simulink model "PLANTA_COMPLETA"  (R2024b)
settings: Solver=FixedStepAuto  StartTime=0.0  StopTime=inf  FixedStep=0.001  MaxStep=0.0005  RelTol=1e-4
undefined symbols (not defined in the file): A_hm, A_tm, at_breakpoints, at_max, b_ha, B_hm, b_ta, B_tm, bcx, bcy, bhd, bhEb, bhm, bt, btd, btm, btw, bwu, C_hm, C_tm, D_hm, D_tm, DiscIntNeverNeededParam, dl_h_ini, dx_l_ini, dx_t_ini, dx_td_ini, dxt_max, dy_l_ini, F01_a_t_max, F01_Ts1, F02_a_h_max, F02_Ts1, F03_a_h_max, F03_a_t_max, F03_dxt_max, F03_Ts1, Fhw_min, g, Hc, ih, it, Jhd_hEb, Jhm_hb, Jtd, Jtm_tb, K_hsa, K_hsia, K_tsa, K_tsia, Kcy, Kd_table, Ke_tita, Ke_w, kp_pos, Kp_table, kp_w, Ktw, kwu, l_breakpoints ... (+30)
libraries: simulink x13, spsEdgeDetectorLib x5, simulink_extras x2, dspsigops x2, vrlib x1, dspstat3 x1
(part 4 of 5)

== system PLANTA_COMPLETA/Nivel 2 - Control Regulatorio + Obs/Observador_Control_Posicion/Fuerzas de tension de cable en Carro ==
  x_td : Inport
  dx_td : Inport  Port=2
  x_t : Inport  Port=3
  dx_t : Inport  Port=4
  Add : Sum  Inputs=+-
  Add1 : Sum  Inputs=+-
  Add2 : Sum
  Gain : Gain  Gain=Ktw
  Gain1 : Gain  Gain=btw
  F_tw : Outport
  wires:
  Add1/1 -> Gain1/1
  Add/1 -> Gain/1
  Gain1/1 -> Add2/2
  x_td/1 -> Add/1
  dx_t/1 -> Add1/2
  dx_td/1 -> Add1/1
  Gain/1 -> Add2/1
  Add2/1 -> F_tw/1
  x_t/1 -> Add/2

== system PLANTA_COMPLETA/Nivel 2 - Control Regulatorio + Obs/Observador_Control_Posicion/Observador ==
  x_td : Inport
  T_tm* : Inport  Port=2
  Discrete-Time Integrator : DiscreteIntegrator  InitialCondition=x_td_ini  SampleTime=T_s2  ICPrevOutput=DiscIntNeverNeededParam  ICPrevScaledInput=DiscIntNeverNeededParam
  Discrete-Time Integrator1 : DiscreteIntegrator  InitialCondition=dx_td_ini  SampleTime=T_s2  ICPrevOutput=DiscIntNeverNeededParam  ICPrevScaledInput=DiscIntNeverNeededParam
  Gain : Gain  Gain=rtd/(Jtd+Jtm_tb*(it)^2)
  Gain1 : Gain  Gain=Ke_tita
  Gain2 : Gain  Gain=Ke_w
  Gain3 : Gain  Gain=it
  Scope : Scope  NumInputPorts=3
  Sum1 : Sum  Inputs=|++
  Sum2 : Sum  Inputs=|++
  Sum3 : Sum  Inputs=+-|
  dx_td_obs : Outport
  wires:
  T_tm*/1 -> Gain3/1
  Gain/1 -> Sum1/1
  Sum1/1 -> Discrete-Time Integrator1/1  "ddx_td_obs"
  x_td/1 -> Scope/1, Sum3/1
  Sum3/1 -> Gain2/1, Gain1/1
  Gain1/1 -> Sum2/2
  Gain2/1 -> Sum1/2
  Sum2/1 -> Scope/3, Discrete-Time Integrator/1, dx_td_obs/1
  Gain3/1 -> Gain/1
  Discrete-Time Integrator/1 -> Scope/2, Sum3/2
  Discrete-Time Integrator1/1 -> Sum2/1

== system PLANTA_COMPLETA/Nivel 2 - Control Regulatorio + Obs/Observador_Control_Posicion/Subsystem ==
  xt_obs : Inport
  xt_ref : Inport  Port=2
  Discrete Derivative : simulink/Discrete/Discrete Derivative  Commented=on  gainval=1.0  ICPrevScaledInput=0.0  OutMin=[]  OutMax=[]  OutDataType=fixdt(1, 16)  OutScaling=2^-10  DoSatur=off
  Gain : Gain  Gain=kp_pos
  Gain1 : Gain  Commented=on  Gain=kp_w
  Sum : Sum  Inputs=|++
  Sum1 : Sum  Inputs=|-+
  dxt_pos : Outport
  wires:
  xt_ref/1 -> Sum1/2
  Sum1/1 -> Discrete Derivative/1, Gain/1
  Gain/1 -> Sum/1  "dxt_pos"
  Gain1/1 -> Sum/2  "dxt_pos"
  Sum/1 -> dxt_pos/1
  xt_obs/1 -> Sum1/1
  Discrete Derivative/1 -> Gain1/1

== system PLANTA_COMPLETA/Nivel 2 - Control Regulatorio + Obs/Observador_Control_Posicion/Traslacion del carro ==
  F_tw : Inport
  F_hw : Inport  Port=2
  theta_l : Inport  Port=3
  Discrete-Time Integrator : DiscreteIntegrator  InitialCondition=dx_t_ini  SampleTime=T_s2  ICPrevOutput=DiscIntNeverNeededParam  ICPrevScaledInput=DiscIntNeverNeededParam
  Discrete-Time Integrator1 : DiscreteIntegrator  InitialCondition=x_t_ini  SampleTime=T_s2  ICPrevOutput=DiscIntNeverNeededParam  ICPrevScaledInput=DiscIntNeverNeededParam
  Gain : Gain  Gain=2
  Gain1 : Gain  Gain=bt
  Gain2 : Gain  Gain=1/Mt
  Product : Product
  Sin : Trigonometry
  Sum : Sum  Inputs=++-
  x_t : Outport
  dx_t : Outport  Port=2
  wires:
  Gain1/1 -> Sum/3
  theta_l/1 -> Sin/1
  Sin/1 -> Product/2
  Sum/1 -> Gain2/1
  F_tw/1 -> Sum/1
  F_hw/1 -> Product/1
  Gain/1 -> Sum/2
  Product/1 -> Gain/1
  Gain2/1 -> Discrete-Time Integrator/1  "ddx_t"
  Discrete-Time Integrator/1 -> Discrete-Time Integrator1/1, Gain1/1, dx_t/1
  Discrete-Time Integrator1/1 -> x_t/1

== system PLANTA_COMPLETA/PLANTA/ACC DE CARRO/Freno ==
  dx_td : Inport
  BRK_t : Inport  Port=2
  Constant : Constant  Value=0
  Gain4 : Gain  Gain=-(btd*it)/rtd
  Saturation : Saturate  UpperLimit=Ttb_Max  LowerLimit=-Ttb_Max
  Switch : Switch  Criteria=u2 ~= 0  SaturateOnIntegerOverflow=off  InputSameDT=off
  T_tb : Outport
  wires:
  Constant/1 -> Switch/1
  BRK_t/1 -> Switch/2
  Saturation/1 -> Switch/3
  Switch/1 -> T_tb/1  "T_tb"
  Gain4/1 -> Saturation/1
  dx_td/1 -> Gain4/1

== system PLANTA_COMPLETA/PLANTA/ACC DE IZAJE/Freno ==
  w_hm : Inport
  BRK_h : Inport  Port=2
  Constant : Constant  Value=0
  Gain5 : Gain  Gain=-bhd
  Saturation : Saturate  UpperLimit=Thb_Max  LowerLimit=-Thb_Max
  Switch : Switch  Criteria=u2 ~= 0  SaturateOnIntegerOverflow=off  InputSameDT=off
  T_hb : Outport
  wires:
  Gain5/1 -> Saturation/1
  BRK_h/1 -> Switch/2
  Saturation/1 -> Switch/3
  Constant/1 -> Switch/1
  w_hm/1 -> Gain5/1
  Switch/1 -> T_hb/1

== system PLANTA_COMPLETA/PLANTA/ACC DE IZAJE/Freno Emergencia ==
  w_hd : Inport
  BRK_hE : Inport  Port=2
  Constant : Constant  Value=0
  Gain5 : Gain  Gain=-bhEb
  Saturation : Saturate  UpperLimit=ThEb_Max  LowerLimit=-ThEb_Max
  Switch : Switch  Criteria=u2 ~= 0  SaturateOnIntegerOverflow=off  InputSameDT=off
  T_hEB : Outport
  wires:
  Gain5/1 -> Saturation/1
  BRK_hE/1 -> Switch/2
  Saturation/1 -> Switch/3
  Constant/1 -> Switch/1
  w_hd/1 -> Gain5/1
  Switch/1 -> T_hEB/1

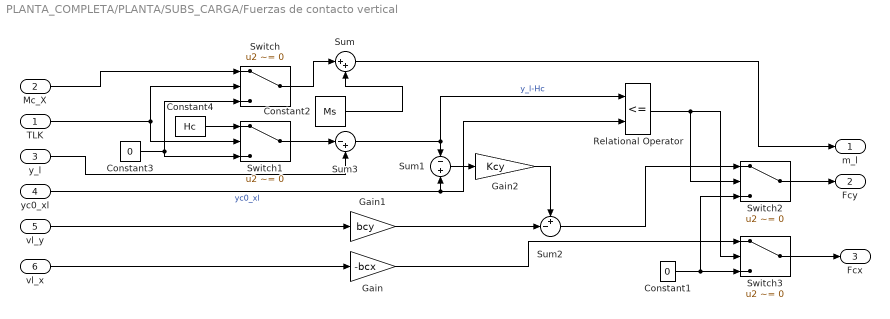
== system PLANTA_COMPLETA/PLANTA/SUBS_CARGA/Fuerzas de contacto vertical ==
  TLK : Inport
  Mc_X : Inport  Port=2
  y_l : Inport  Port=3
  yc0_xl : Inport  Port=4
  vl_y : Inport  Port=5
  vl_x : Inport  Port=6
  Constant1 : Constant  Value=0
  Constant2 : Constant  Value=Ms
  Constant3 : Constant  Value=0
  Constant4 : Constant  Value=Hc
  Gain : Gain  Gain=-bcx
  Gain1 : Gain  Gain=bcy
  Gain2 : Gain  Gain=Kcy
  Relational Operator : RelationalOperator  Operator=<=  OutDataTypeStr=boolean  RndMeth=Simplest  InputSameDT=off
  Sum : Sum  Inputs=|++
  Sum1 : Sum  Inputs=-|+
  Sum2 : Sum  Inputs=+-|
  Sum3 : Sum  Inputs=|-+
  Switch{,1..3} (4 alike) : Switch  Criteria=u2 ~= 0  SaturateOnIntegerOverflow=off  InputSameDT=off
  m_l : Outport
  Fcy : Outport  Port=2
  Fcx : Outport  Port=3
  wires:
  TLK/1 -> Switch/2, Switch1/2
  Gain1/1 -> Sum2/2
  Switch/1 -> Sum/1
  Constant3/1 -> Switch1/3, Switch/3
  Constant2/1 -> Sum/2
  Sum2/1 -> Switch2/1
  vl_y/1 -> Gain1/1
  Gain/1 -> Switch3/1
  Constant4/1 -> Switch1/1
  vl_x/1 -> Gain/1
  Gain2/1 -> Sum2/1
  Sum1/1 -> Gain2/1
  Sum/1 -> m_l/1
  Mc_X/1 -> Switch/1
  Constant1/1 -> Switch3/3, Switch2/3
  Relational Operator/1 -> Switch3/2, Switch2/2
  Sum3/1 -> Sum1/1, Relational Operator/1  "y_l-Hc"
  Switch1/1 -> Sum3/1
  y_l/1 -> Sum3/2
  Switch2/1 -> Fcy/1
  Switch3/1 -> Fcx/1
  yc0_xl/1 -> Relational Operator/2, Sum1/2  "yc0_xl"

== matlab function PLANTA_COMPLETA/PLANTA/PERFIL_OBSTACULOS/sensor ==
  data: y0_array input; distancia output; index input; Yt0 parameter
function distancia= mideDistancia(y0_array,index, Yt0)
distancia = Yt0-y0_array(index);

== matlab function PLANTA_COMPLETA/PLANTA/Altura perfil obstaculos (A partir de posicion x_l)/Calculo ==
  data: y0_array input; yc0_xt output; index input
function yc0_xt= calcula_y0(y0_array,index)

if (index>0 && index<=32)
    yc0_xt =y0_array(index);
else
    yc0_xt=0;    
end

== stateflow chart PLANTA_COMPLETA/Nivel 1 - Control Supervisor ==
  state PERFIL_DE_OBSTACULOS [parallel]
    entry:
    num_index = floor(80/Wc);
    Y_perfil = zeros(1,num_index,'double');
    during:
    %xtd = theta_mt*pulsos_x_rev*dist_x_pulso*(1/100);
    xtd_lidar = (xtd+30)+3;
    index = floor(xtd_lidar/Wc);
    Y_c0_read = yc0_xt;
    if index>0 && index<=32
    Y_perfil(index) = Y_c0_read;
    end
    settings: executionOrder=2
  state OFF [parallel]
    settings: executionOrder=1
    state EMERGENCIA
      entry:
      %Cuando el control supervisor entra en esta de emergencia, cede
      %el control al Nivel 0 hasta retomar el estado normal
      dxt_ref=0;
      dlh_ref=0;
      ddxt_ref=0;
    state ON
      entry:
      dxt_ref_ant = 0;
      dlh_ref_ant = 0;
      dxt_ref = 0;
      dlh_ref = 0;
      ddxt_ref = 0;
      state DETECCION_ESTADOS [parallel]
        settings: executionOrder=1
        state TWISTLOCKS [parallel]
          settings: executionOrder=1
          state VERIFICAR
          state ACT_TLK
            entry:
            TLK=1;
            c=-ceil((xtd+30)/Wc);
            during:
            y_real=45-(lh+Hc);
          state DES_TLK
            entry:
            TLK=0;
            c=ceil((xtd+30)/Wc);
            during:
            y_real=45-lh;
          (default) -> VERIFICAR
          VERIFICAR -> ACT_TLK [order 2] : [TLK_act==1]
          VERIFICAR -> DES_TLK [order 1] : [TLK_act==0]
          ACT_TLK -> DES_TLK : [TLK_act==0 && op_mode==1 && cable_tenso==0]
          DES_TLK -> ACT_TLK : [TLK_act==1 && op_mode==1 && cable_tenso==0]
        state FRENOS [parallel]
          settings: executionOrder=2
          state FRENO_IZAJE [parallel]
            settings: executionOrder=1
            state FRENO_IZAJE_OFF
              entry:
              BRK_h=1;
              parar_izaje=0;
            state FRENO_IZAJE_ON
              entry:
              BRK_h=0;
              parar_izaje=1;
            (default) -> FRENO_IZAJE_ON
            FRENO_IZAJE_OFF -> FRENO_IZAJE_ON : [(abs(whm)<=whm_min && (abs(whm) < abs(whm_ant)-(whm_min*0.01)))]
            FRENO_IZAJE_ON -> FRENO_IZAJE_OFF : [abs(Thm_disp) && (abs(dlh_ref)>0.1 || dlh_ref_man~=0) && after(0.2,sec)]
          state FRENO_CARRO [parallel]
            settings: executionOrder=2
            state FRENO_CARRO_OFF
              entry:
              BRK_t=1;
              parar_carro=0;
            state FRENO_CARRO_ON
              entry:
              BRK_t=0;
              parar_carro=1;
            (default) -> FRENO_CARRO_ON
            FRENO_CARRO_OFF -> FRENO_CARRO_ON : [(abs(wtm)<=wtm_min && (abs(wtm)<abs(wtm_ant)-wtm_min*0.01))]
            FRENO_CARRO_ON -> FRENO_CARRO_OFF : [abs(Ttm_disp) && (abs(dxt_ref)>0.1 || dxt_ref_man~=0) && after(0.2,sec)]
        state FINALES [parallel]
          settings: executionOrder=3
          state FIN_CARRERA_CARRO [parallel]
            settings: executionOrder=1
            state PARAR_CARRO
              entry:
              op_mode=1;
              parar_carro=1;
            state MOVER_CARRO
              entry:
              parar_carro=0;
            (default) -> MOVER_CARRO
            OFF.ON.DETECCION_ESTADOS.FINALES.FIN_CARRERA_CARRO.PARAR_CARRO -> MOVER_CARRO : [xt_ref<0 && dxt_ref>0 || xt_ref>0 && dxt_ref<0]
            MOVER_CARRO -> OFF.ON.DETECCION_ESTADOS.FINALES.FIN_CARRERA_CARRO.PARAR_CARRO : [(FC_DER==1 && dxt_ref>0) || (FC_IZQ==1 && dxt_ref<0)]
          state FIN_CARRERA_IZAJE [parallel]
            settings: executionOrder=2
            state PARAR_CARGA
              entry:
              op_mode=1;
              parar_carga=1;
            state MOVER_CARGA
              entry:
              parar_carga=0;
            (default) -> MOVER_CARGA
            PARAR_CARGA -> MOVER_CARGA : [whm<=0.3]
            MOVER_CARGA -> PARAR_CARGA : [(FC_SUP==1 && dlh_ref>0) || (FC_INF && dlh_ref<0)]
        state CONTROL_BALANCEO [parallel]
          settings: executionOrder=4
          state BALANCEO_ON
            entry:
            bal_control=1;
          state BALANCEO_OFF
            entry:
            bal_control=0;
          (default) -> BALANCEO_ON
          BALANCEO_ON -> BALANCEO_OFF : [~balanceo_on || falla_E~=0]
          BALANCEO_OFF -> BALANCEO_ON : [balanceo_on]
        state TENSION_CABLE_IZAJE [parallel]
          settings: executionOrder=5
          state TENSO
            entry:
            cable_tenso=1;
          state FLOJO
            entry:
            cable_tenso=0;
          (default) -> TENSO
          TENSO -> FLOJO : [Fhw < Fhw_min]
          FLOJO -> TENSO : [Fhw >= Fhw_min]
      state SUPERVISION [parallel]
        settings: executionOrder=2
        state ENCLAVAMIENTO_MASA [parallel]
          settings: executionOrder=3
          state INICIO
            entry:
            Ml_estimada=15000;
            dlh_max_estimada=3;
            aceptar_carga=0;
          state ESTABILIZACION
            entry:
            contador_fuerza_estable = 0;
            fuerza_estabilizada=0;
            N_estable=50;
            Fhw_ant=Fhw;
            during:
            if(abs(Fhw-Fhw_ant)<1000)
            contador_fuerza_estable = contador_fuerza_estable + 1;
            else
            contador_fuerza_estable = 0;
            end
            if contador_fuerza_estable >= N_estable
            fuerza_estabilizada = 1;
            else
            fuerza_estabilizada = 0;
            end
            Fhw_ant = Fhw;
          state ACEPTAR_CARGA
            entry:
            Ml_estimada=Ml;
            dlh_max_estimada=dlh_max;
            aceptar_carga=1;
          (default) -> INICIO
          ACEPTAR_CARGA -> INICIO : [TLK==0]
          INICIO -> ESTABILIZACION : [TLK==1 && cable_tenso==1]
          ESTABILIZACION -> ACEPTAR_CARGA : [fuerza_estabilizada==1]
        state DETECION_SOBRECARGA [parallel]
          settings: executionOrder=1
          state NORMAL
            entry:
            sobrecarga=0;
          state SOBRECARGA
            entry:
            sobrecarga=1;
          (default) -> NORMAL
          NORMAL -> OFF.ON.SUPERVISION.DETECION_SOBRECARGA.SOBRECARGA : [cable_tenso && ((Ml_estimada-Ms) > Mc_max) && aceptar_carga==1]
          OFF.ON.SUPERVISION.DETECION_SOBRECARGA.SOBRECARGA -> NORMAL : [cable_tenso == 0]
        state CONTROL_SOBREVELOCIDAD [parallel]
          settings: executionOrder=2
          state ON
            state SP_CARRO [parallel]
              settings: executionOrder=1
              state CARRO
                during:
                dxt_sp=dxt_ref_man;
              state SOBRE_dxt_MIN
                entry:
                dxt_sp=-dxt_max;
              state SOBRE_dxt_MAX
                entry:
                dxt_sp=dxt_max;
              (default) -> OFF.ON.SUPERVISION.CONTROL_SOBREVELOCIDAD.ON.SP_CARRO.CARRO
              SOBRE_dxt_MIN -> OFF.ON.SUPERVISION.CONTROL_SOBREVELOCIDAD.ON.SP_CARRO.CARRO : [dxt_ref_man >= -dxt_max]
              OFF.ON.SUPERVISION.CONTROL_SOBREVELOCIDAD.ON.SP_CARRO.CARRO -> SOBRE_dxt_MIN [order 2] : [dxt_ref_man < -dxt_max]
              SOBRE_dxt_MAX -> OFF.ON.SUPERVISION.CONTROL_SOBREVELOCIDAD.ON.SP_CARRO.CARRO : [dxt_ref_man <= dxt_max]
              OFF.ON.SUPERVISION.CONTROL_SOBREVELOCIDAD.ON.SP_CARRO.CARRO -> SOBRE_dxt_MAX [order 1] : [dxt_ref_man > dxt_max]
            state SP_IZAJE [parallel]
              settings: executionOrder=2
              state IZAJE
                during:
                dlh_sp=dlh_ref_man;
              state SOBRE_dhl_MIN
                entry:
                dlh_sp=-dlh_max_estimada
              state SOBRE_dhl_MAX
                entry:
                dlh_sp=dlh_max_estimada
              (default) -> OFF.ON.SUPERVISION.CONTROL_SOBREVELOCIDAD.ON.SP_IZAJE.IZAJE
              SOBRE_dhl_MIN -> OFF.ON.SUPERVISION.CONTROL_SOBREVELOCIDAD.ON.SP_IZAJE.IZAJE : [dlh_ref_man >= -dlh_max_estimada]
              OFF.ON.SUPERVISION.CONTROL_SOBREVELOCIDAD.ON.SP_IZAJE.IZAJE -> SOBRE_dhl_MIN [order 2] : [dlh_ref_man < -dlh_max_estimada]
              SOBRE_dhl_MAX -> OFF.ON.SUPERVISION.CONTROL_SOBREVELOCIDAD.ON.SP_IZAJE.IZAJE : [dlh_ref_man <= dlh_max_estimada]
              OFF.ON.SUPERVISION.CONTROL_SOBREVELOCIDAD.ON.SP_IZAJE.IZAJE -> SOBRE_dhl_MAX [order 1] : [dlh_ref_man > dlh_max_estimada]
          (default) -> OFF.ON.SUPERVISION.CONTROL_SOBREVELOCIDAD.ON
      state OPERACION [parallel]
        entry:
        xt_ref = xtd;
        lh_ref = 20;
        settings: executionOrder=3
        state MODO_MANUAL
          entry:
          op_mode=1;
          state CARRO [parallel]
            settings: executionOrder=1
            state CARRO_ON
              during:
              [xt_ref, dxt_ref, ddxt_ref]=limitar_aceleracion_x(dxt_sp,xtd);
            state DIST_FDC_IZQ
              during:
              [xt_ref, dxt_ref, ddxt_ref]=limitar_aceleracion_x(dxt_sp*(30+xtd)/11,xtd);
            state PARAR_CARRO
              entry:
              dxt_ref=0;
            state DIST_FDC_DER
              during:
              [xt_ref, dxt_ref, ddxt_ref]=limitar_aceleracion_x(dxt_sp*(50-xtd)/11,xtd);
            state SOBRECARGA
              entry:
              dxt_ref=0;
            (default) -> CARRO_ON
            CARRO_ON -> DIST_FDC_IZQ [order 1] : [xtd <= -19  && dxt_sp < 0 && parar_carro == 0]
            CARRO_ON -> OFF.ON.OPERACION.MODO_MANUAL.CARRO.PARAR_CARRO [order 4] : [parar_carro]
            DIST_FDC_IZQ -> CARRO_ON : [(xtd > -19 && dxt_sp > 0) || parar_carro == 1 ]
            OFF.ON.OPERACION.MODO_MANUAL.CARRO.PARAR_CARRO -> CARRO_ON : [~parar_carro]
            CARRO_ON -> DIST_FDC_DER [order 2] : [xtd >= 39  && dxt_sp > 0 && parar_carro == 0]
            CARRO_ON -> OFF.ON.OPERACION.MODO_MANUAL.CARRO.SOBRECARGA [order 3] : [sobrecarga]
            OFF.ON.OPERACION.MODO_MANUAL.CARRO.SOBRECARGA -> CARRO_ON : [~sobrecarga]
            DIST_FDC_DER -> CARRO_ON : [(xtd < 39 && dxt_sp < 0) || parar_carro == 1 ]
          state IZAJE [parallel]
            settings: executionOrder=2
            state IZAJE_ON
              during:
              dlh_ref=limitar_aceleracion_y(dlh_sp,0);
            state DIST_FDC_SUP
              during:
              dlh_ref=limitar_aceleracion_y(dlh_sp*(lh-5)/7,0);
            state PARAR_IZAJE
              entry:
              dlh_ref=0;
            state DIST_FDC_INF
              during:
              dlh_ref=limitar_aceleracion_y(dlh_sp*(65-lh)/10,0);
            state SOBRECARGA
              during:
              if (dlh_sp>=0)
              dlh_ref=dlh_sp*0.1;
              else
              end
            state ALTURA_BAJA
              during:
              %Nos elevamos a aceleracion despreciable
              dlh_ref=limitar_aceleracion_y(dlh_ref_man,0)*0.08;
              exit:
              limitar_aceleracion_y(dlh_ref,1);
            (default) -> IZAJE_ON
            IZAJE_ON -> DIST_FDC_SUP [order 1] : [lh <= 12 && dlh_sp < 0 && parar_izaje == 0]
            DIST_FDC_SUP -> IZAJE_ON : [(lh > 12 && dlh_sp > 0) || parar_izaje == 1 ]
            PARAR_IZAJE -> IZAJE_ON : [~parar_izaje]
            IZAJE_ON -> DIST_FDC_INF [order 2] : [lh >= 55 && dlh_sp > 0 && parar_izaje == 0]
            IZAJE_ON -> PARAR_IZAJE [order 3] : [parar_izaje]
            DIST_FDC_INF -> IZAJE_ON : [(lh < 55 && dlh_sp > 0) && parar_izaje == 1]
            OFF.ON.OPERACION.MODO_MANUAL.IZAJE.SOBRECARGA -> IZAJE_ON : [~sobrecarga]
            IZAJE_ON -> ALTURA_BAJA [order 5] : [TLK==1 && cable_tenso==1 && aceptar_carga == 0]
            IZAJE_ON -> OFF.ON.OPERACION.MODO_MANUAL.IZAJE.SOBRECARGA [order 4] : [sobrecarga]
            ALTURA_BAJA -> IZAJE_ON : [aceptar_carga == 1]
        state MODO_AUTOMATICO
          entry:
          % 1. Configuración Inicial
          op_mode = 0; % Modo Automático
          it = 1;      % Índice de tiempo (iterador)
          % 2. Definir parámetros para la función
          % Asegúrate de que v_max, etc., sean variables conocidas en el workspace o Data Store
          x_inicial = xtd;        % Posición actual real (no la deseada anterior)
          x_final = destino;
          y_inicial = y_real;
          % 3. Generar la trayectoria COMPLETA una sola vez al entrar
          % La función devuelve una matriz 'consignas' de tamaño 6 x N
          % Fila 1: Referencia X, Fila 2: Referencia lh
          trayectoria = gen_coords(Y_c0, dlh_max_estimada, xtd, destino,y_real);
          % Obtener la longitud de la maniobra
          dims = size(trayectoria);
          % Capturar el tiempo exacto de inicio de la maniobra
          % 't_sim' debe ser una entrada al chart proveniente del bloque 'Clock' de Simulink
          it_ultimo=0;
          it_max = dims(2);
          during:
          % Asignación de referencias (Igual que antes)
          if(it<it_max)
          xt_ref  = trayectoria(1, it);
          lh_ref  = trayectoria(2, it);
          dxt_ref = trayectoria(3, it);
          dlh_ref = trayectoria(4, it);
          ddxt_ref = trayectoria(5, it);
          end
          it=it+1;
          exit: % Condición de salida (Fin de trayectoria)
          dxt_ref_ant = dxt_ref;
          dlh_ref_ant = dlh_ref;
          ddxt_ref_ant = ddxt_ref;
        (default) -> MODO_MANUAL
        MODO_AUTOMATICO -> MODO_MANUAL [order 2] : [dxt_ref_man ~= 0 || dlh_ref_man ~= 0]
        MODO_AUTOMATICO -> MODO_MANUAL [order 3] : [((y_real < (yc0_xt+4)) && abs(tita_l)<=tita_l_max_estable) && abs(wtm)<=wtm_min ]
        MODO_MANUAL -> MODO_AUTOMATICO : [(y_real >= (yc0_xt+4)) && (dxt_ref_man == 0 && dlh_ref_man == 0) && (~parar_carro)]
        MODO_AUTOMATICO -> MODO_MANUAL [order 1] : [FC_DER || FC_IZQ || FC_SUP || FC_INF]
      state VIVO [parallel]
        settings: executionOrder=4
        state WAIT
          entry:
          alive=0;
        state TALK
          entry:
          alive=1;
        (default) -> WAIT
        WAIT -> TALK : [after(500,msec)]
        TALK -> WAIT : [after(20,msec)]
    (default) -> OFF.ON
    EMERGENCIA -> OFF.ON : [~falla_E]
    OFF.ON -> EMERGENCIA : [falla_E]
  data: xt_manual function_output; dx_manual function_input; vel_maxima_x function_output; F01_a_t_max parameter; F01_Ts1 parameter; a_maxima_x function_output; x_actual function_input; dy_manual function_input; v_maxima_y function_output; estado function_input; at_max parameter; F02_Ts1 parameter; F02_a_h_max parameter; perfil_modif function_input; v_max_izaje function_input; x_inicio function_input; x_destino function_input; y_inicio function_input; F03_Ts1 parameter; consignas function_output; F03_dxt_max parameter; F03_a_t_max parameter; xx_c0 parameter; F03_a_h_max parameter; dxt_ref output; dlh_ref output; Mc_max parameter double; y_inicial local double size=1; Fhw input; Fhw_min parameter; Ml input; FC_SUP input; FC_INF input; FC_IZQ input; FC_DER input; xtd input; x_inicial local size=1; x_fin_consigna local =0; pos_ref local size=[2 400000]; parametros local; num_index local; it_fin local int16 =20000; it local; index local; cable_tenso local double; Y_c0_read local; TLK output =0; Kp local; xtd_lidar local; c output =2000; bal_control output size=1; Y_perfil local double size=[1, floor(80/Wc)]; whm input; whm_ant input; wtm input; wtm_ant input; whm_min parameter; wtm_min parameter; lh input; falla_E input int8; dlh_max input; dlh_ref_man input; dxt_ref_man input; BRK_h output; BRK_t output; destino input; balanceo_on input; TLK_act input; Wc parameter; T_s1 parameter; parar_izaje local; parar_carro local; parar_carga local; alive output double =1; emergency local; dxt_max parameter; dxt_sp local =0; dlh_sp local =0; tol_lh local; tol_x local; lh_max_permitida local; i local; Y_c0 input; yc0_xt input; dims local; trayectoria local size=[5 400000]; x_final local; it_max local; v_h_max local; it_calculado local; t_inicio local; pausa_global local; it_ultimo local; dtsimu local; Hc parameter; y_real local =0; dxt_ref_ant local; dlh_ref_ant local; Ttm_disp input =1; Thm_disp input =1; rhd parameter; ih parameter; aceptar_carga local; fuerza_estabilizada local; contador_fuerza_estable local; N_estable local; Fhw_ant local; Ms parameter; Ml_estimada output =0; ddxt_ref output; xt_ref output; lh_ref output; ddxt_ref_ant local; tita_l input; tita_l_max_estable parameter; BRK_hE local; dlh_max_estimada output; sobrecarga output double =0; op_mode output double; dxt_ref_prev local
  function [xt_manual, vel_maxima_x, a_maxima_x] = limitar_aceleracion_x(dx_manual,x_actual):
    | function [xt_manual, vel_maxima_x, a_maxima_x] = limitar_aceleracion_x(dx_manual,x_actual)
    | 
    | persistent dx_tref_manual_ant
    | persistent dx_tref_manual_ant_2
    | 
    | %x0 = xt_ref;
    | 
    | %Asignacion de variables externas
    | a_t_max=F01_a_t_max;
    | tiempo_muestreo=F01_Ts1;
    | 
    | if isempty(dx_tref_manual_ant)
    |     dx_tref_manual_ant=0;
    | end
    | if isempty(dx_tref_manual_ant_2)
    |     dx_tref_manual_ant_2=0;
    | end
    | if abs(dx_manual)>=abs(dx_tref_manual_ant)
    |     if dx_manual>0
    |         v_max=a_t_max*tiempo_muestreo+dx_tref_manual_ant;
    |         if dx_manual>v_max
    |              vel_maxima_x=v_max;
    |         else 
    |             vel_maxima_x=dx_manual;
    |         end
    | 
    |     else 
    |         v_max=-a_t_max*tiempo_muestreo+dx_tref_manual_ant;
    |         if dx_manual<v_max
    |             vel_maxima_x=v_max;
    |         else 
    |             vel_maxima_x=dx_manual;
    |         end
    |     end
    | else
    |     if dx_manual<dx_tref_manual_ant
    |         v_max=-a_t_max*tiempo_muestreo+dx_tref_manual_ant;
    |         if dx_manual<v_max
    |              vel_maxima_x=v_max;
    |         else 
    |             vel_maxima_x=dx_manual;
    |         end
    | 
    |     else 
    |         v_max=a_t_max*tiempo_muestreo+dx_tref_manual_ant;
    |         if dx_manual>v_max
    |             vel_maxima_x=v_max;
    |         else 
    |             vel_maxima_x=dx_manual;
    |         end
    |     end
    | end
    | a_maxima_x = (vel_maxima_x-dx_tref_manual_ant_2)/2*tiempo_muestreo;
    | %xt_manual = x0+(dx_tref_manual_ant_2+4*dx_tref_manual_ant+vel_maxima_x)*tiempo_muestreo/3;
    | xt_manual = x_actual;
    | dx_tref_manual_ant_2=dx_tref_manual_ant;
    | dx_tref_manual_ant=vel_maxima_x;
    | end
  function v_maxima_y = limitar_aceleracion_y(dy_manual,estado):
    | function v_maxima_y = limitar_aceleracion_y(dy_manual,estado)
    | 
    | persistent dy_href_manual_ant
    | 
    | % Asignacion de variables externas
    | a_h_max = F02_a_h_max;
    | tiempo_muestreo = F02_Ts1;
    | 
    | if isempty(dy_href_manual_ant)
    |     dy_href_manual_ant = 0;
    | end
    | 
    | if estado == 0
    | 
    |     % Detectar cambio de signo
    |     if dy_manual * dy_href_manual_ant < 0
    |         dy_href_manual_ant = 0;
    |     end
    | 
    |     delta = dy_manual - dy_href_manual_ant;
    |     delta_max = a_h_max * tiempo_muestreo;
    | 
    |     if delta > delta_max
    |         delta = delta_max;
    |     elseif delta < -delta_max
    |         delta = -delta_max;
    |     end
    | 
    |     v_maxima_y = dy_href_manual_ant + delta;
    | 
    |     dy_href_manual_ant = v_maxima_y;
    | 
    | else
    | 
    |     v_maxima_y = dy_manual;
    |     dy_href_manual_ant = dy_manual;
    | 
    | end
    | 
    | end
    | % function v_maxima_y = limitar_aceleracion_y(dy_manual,estado)
    | % 
    | % persistent dy_href_manual_ant
    | % 
    | % Asignacion de variables externas
    | % a_h_max=F02_a_h_max;
    | % tiempo_muestreo=F02_Ts1;
    | % 
    | % if isempty(dy_href_manual_ant)
    | %     dy_href_manual_ant=0;
    | % end
    | % if estado==0
    | %     if abs(dy_manual)>=abs(dy_href_manual_ant)
    | %         if dy_manual>0
    | %             v_max=a_h_max*tiempo_muestreo+dy_href_manual_ant;
    | %             if dy_manual>v_max
    | %                 v_maxima_y=v_max;
    | %             else 
    | %                 v_maxima_y=dy_manual;
    | %             end
    | % 
    | %         else 
    | %             v_max=-a_h_max*tiempo_muestreo+dy_href_manual_ant;
    | %             if dy_manual<v_max
    | %                 v_maxima_y=v_max;
    | %             else 
    | %                 v_maxima_y=dy_manual;
    | %             end
    | %         end
    | %     else
    | %         if dy_manual<dy_href_manual_ant
    | %             v_max=-a_h_max*tiempo_muestreo+dy_href_manual_ant;
    | %             if dy_manual<v_max
    | %                  v_maxima_y=v_max;
    | %             else 
    | %                 v_maxima_y=dy_manual;
    | %             end
    | % 
    | %         else 
    | %             v_max=a_h_max*tiempo_muestreo+dy_href_manual_ant;
    | %             if dy_manual>v_max
    | %                 v_maxima_y=v_max;
    | %             else 
    | %                 v_maxima_y=dy_manual;
    | %             end
    | %         end
    | %     end
    | %     dy_href_manual_ant=v_maxima_y;
    | % else 
    | %     dy_href_manual_ant=dy_manual;
    | % end
    | % end
  function consignas = gen_coords(perfil_modif,v_max_izaje,x_inicio,x_destino,y_inicio):
    | % function consignas = gen_coords(Y_c0_vector_modif,v_max_izaje_valor,x_t_inicial,x_t_final,y_l_inicial)
    | % %consignas: Matriz 2xn con referencias en x y lh muestreadas
    | % %Y_c0_vector_modif: Perfil de obstaculos (altura)
    | % %v_max_izaje_valor: Vel maxima de izaje (en eje vertical)
    | % %x_t_inicial, x_t_final: Posicion inicial y final en X
    | % %y_l_inicial: Altura inicial (y, no lh)
    | % %sample_time: periodo de muestreo
    | % 
    | % %Asignación de variables externas
    | % a_h_max=F03_a_h_max; %Aceleracion max de izaje
    | % a_t_max=F03_a_t_max; %Aceleracion max de carro
    | % v_t_max=F03_dxt_max; %Velocidad max carro
    | % tiempo_muestreo=F03_Ts1; %Muestreo sistema de control N1
    | % 
    | % % Índices del perfil y límites de seguridad
    | % index_inicial = round((x_t_inicial+30)/2.44);
    | % index_final   = round((x_t_final+30)/2.44);
    | % index_inicial = max(1, min(index_inicial, length(Y_c0_vector_modif)));
    | % index_final   = max(1, min(index_final, length(Y_c0_vector_modif)));
    | % 
    | % % Parámetros locales
    | % x_inicial = x_t_inicial;
    | % x_final   = x_t_final;
    | % y_inicial = y_l_inicial;     % altura inicial (y)
    | % v_h_max   = v_max_izaje_valor;
    | % margen_seg = 3;              
    | % 
    | % % Obtenemos el perfil de obstáculos
    | % if index_inicial <= index_final
    | %     Y_c0_tramo = Y_c0_vector_modif(index_inicial:index_final);
    | % else
    | %     Y_c0_tramo = Y_c0_vector_modif(index_inicial:-1:index_final);
    | % end
    | % 
    | % % PARCHE 1: Forzar vector fila. Evita que la matemática explote al ir a la izquierda
    | % Y_c0_tramo = reshape(Y_c0_tramo, 1, []);
    | % 
    | % % Construcción de la Envolvente de Seguridad
    | % y_req_tramo = Y_c0_tramo + margen_seg;
    | % x_tramo = linspace(x_inicial, x_final, length(y_req_tramo));
    | % y_final = Y_c0_vector_modif(index_final) + margen_seg;  
    | % 
    | % % 1. Encontrar el pico 
    | % [y_peak_obs, idx_peak] = max(y_req_tramo);
    | % x_peak = x_tramo(idx_peak);
    | % 
    | % % PARCHE 2: Evitar el valle (Dip) si los obstáculos son más bajos que el inicio/fin
    | % y_peak = max([y_peak_obs, y_inicial, y_final]);
    | % 
    | % % Saturaciones de seguridad
    | % y_peak  = min(max(y_peak, 0), 45);
    | % y_final = min(max(y_final, 0), 45);
    | % 
    | % % 2. Ancla izquierda
    | % y_left_anchor = y_req_tramo(1);
    | % % PARCHE 3: Evitar división por cero si el pico está en el inicio
    | % if abs(x_peak - x_inicial) > 1e-3 
    | %     for i = 1:idx_peak-1
    | %         t_i = (x_tramo(i) - x_inicial) / (x_peak - x_inicial);
    | %         if t_i < 1 && t_i >= 0
    | %             req_anchor = (y_req_tramo(i) - y_peak * t_i) / (1 - t_i);
    | %             if req_anchor > y_left_anchor
    | %                 y_left_anchor = req_anchor; 
    | %             end
    | %         end
    | %     end
    | % end
    | % y_left_anchor = min(max([y_left_anchor, y_inicial, 0]), 45);
    | % 
    | % % 3. Ancla derecha
    | % y_right_anchor = y_req_tramo(end);
    | % % PARCHE 3: Evitar división por cero si el pico está en el fin
    | % if abs(x_final - x_peak) > 1e-3
    | %     for i = idx_peak+1:length(y_req_tramo)
    | %         u_i = (x_tramo(i) - x_peak) / (x_final - x_peak);
    | %         if u_i > 0 && u_i <= 1
    | %             req_anchor = (y_req_tramo(i) - y_peak) / u_i + y_peak;
    | %             if req_anchor > y_right_anchor
    | %                 y_right_anchor = req_anchor; 
    | %             end
    | %         end
    | %     end
    | % end
    | % y_right_anchor = min(max([y_right_anchor, y_final, 0]), 45);
    | % 
    | % % 4. Waypoints base
    | % epsilon = 1e-5; % 0.01 milímetros, despreciable para el motor
    | % ptos_x = [x_inicial, x_inicial + epsilon, x_peak, x_final - epsilon, x_final];
    | % ptos_y = [y_inicial, y_left_anchor, y_peak, y_right_anchor, y_final];
    | % 
    | % % 5. Remover waypoints duplicados (El método original fluido)
    | % wpts_xy  = [ptos_x; ptos_y];
    | % idx_keep = [true, sum(abs(diff(wpts_xy, 1, 2))) > 1e-3];
    | % ptos_x   = ptos_x(idx_keep);
    | % ptos_y   = ptos_y(idx_keep);
    | % 
    | % % Convertir a lh
    | % ptos_y = 45 - ptos_y;
    | % 
    | % %||=================================================||
    | % %||            CÁLCULO DE TIEMPOS                   ||
    | % %||=================================================||
    | % delta_x = diff(ptos_x);
    | % delta_y = diff(ptos_y);
    | % 
    | % t = zeros(1, length(ptos_x));
    | % t(1) = 0;
    | % for i = 2:length(ptos_x)
    | %     t_h = abs(delta_y(i-1))/v_h_max;
    | %     t_t = abs(delta_x(i-1))/v_t_max;
    | %     t(i) = t(i-1) + max(t_h, t_t);
    | %     if t(i) == t(i-1)
    | %         t(i) = t(i-1) + 0.5;
    | %     end
    | % end
    | % 
    | % % Interpolación suave (Original pero garantizando que no se pierda el final)
    | % %tiempo_nuevo = unique([0:0.5:t(end), t(end)]);
    | % %ptos_xx = interp1(t,ptos_x,tiempo_nuevo,'linear');
    | % %ptos_yy = interp1(t,ptos_y,tiempo_nuevo,'linear');
    | % wpts = [ptos_x; ptos_y];
    | % 
    | % vellim   = 0.9*[-v_t_max v_t_max; -v_h_max v_h_max];
    | % accellim = 0.9*[-a_t_max a_t_max; -a_h_max a_h_max];
    | % 
    | % [q,qd,qdd,tvec] = contopptraj(wpts,vellim,accellim); 
    | % 
    | % tiempo_consig = 0:tiempo_muestreo:tvec(end);
    | % consignas = zeros(5,length(tiempo_consig));
    | % consignas(1,:) = interp1(tvec,q(1,:),tiempo_consig,'pchip'); %xt_ref
    | % consignas(2,:) = interp1(tvec,q(2,:),tiempo_consig,'pchip'); %lh_ref
    | % consignas(3,:) = interp1(tvec,qd(1,:),tiempo_consig,'pchip'); %dxt_ref
    | % consignas(4,:) = interp1(tvec,qd(2,:),tiempo_consig,'pchip'); %dlh_ref
    | % consignas(5,:) = interp1(tvec,qdd(1,:),tiempo_consig,'linear'); %ddxt_ref
    | % 
    | % end
    | 
    | function consignas = gen_coords(perfil_modif,v_max_izaje,x_inicio,x_destino,y_inicio)
    | %consignas: Matriz 2xn con referencias en x y lh muestreadas
    | %Y_c0_vector_modif: Perfil de obstaculos (altura)
    | %v_max_izaje_valor: Vel maxima de izaje (en eje vertical)
    | %x_t_inicial, x_t_final: Posicion inicial y final en X
    | %y_l_inicial: Altura inicial (y, no lh)
    | %sample_time: periodo de muestreo
    | 
    | %% Inicio Funcion
    | %Asignación de variables externas
    | ah_max=F03_a_h_max; %Aceleracion max de izaje
    | at_max=F03_a_t_max; %Aceleracion max de carro
    | vt_max=F03_dxt_max; %Velocidad max carro
    | Ts=0.02; %Muestreo sistema de control N1
    | 
    | % Parámetros locales
    | x_ini = x_inicio
    | x_fin = x_destino
    | y_ini = y_inicio    % altura inicial (y)
    | vh_max = v_max_izaje;
    | margen_seg = 3;        
    | perfil_seg = perfil_modif+margen_seg;
    | 
    | % Índices del perfil y límites de seguridad
    | idx_ini = round((x_ini+30)/2.44);
    | idx_fin = round((x_fin+30)/2.44);
    | idx_ini = max(1, min(idx_ini, length(perfil_seg)));
    | length(idx_ini)
    | idx_fin   = max(1, min(idx_fin, length(perfil_seg)));
    | length(idx_fin)
    | y_fin = perfil_seg(idx_fin);
    | 
    | %% Obtenemos el perfil de obstáculos en el tramo
    | 
    | % Determinamos lo indices i_min e i_max de menor a mayor
    | i_min = min(idx_ini, idx_fin);
    | i_max = max(idx_ini, idx_fin);
    | 
    | % Extraemos el perfil seguro y perfil de obstaculos siempre de menor a
    | % mayor para evitar que se asigne vacio
    | perfil = perfil_seg;
    | perfil_rec = perfil_seg(i_min:i_max);
    | 
    | %Si el movimiento de izquierda a derecha, se mantiene la asignacion
    | 
    | %Si el movimiento es de derecha a izquierda, se invierte el recorrido de
    | %los vectores
    | if idx_ini > idx_fin
    |     perfil = flip(perfil)
    |     perfil_rec = flip(perfil_rec)
    | end
    | 
    | %% Trayecto 1: Primer parte de la trayectoria
    | %Revisamos alrededores para evitar colisiones
    | if (y_inicio <= perfil(idx_ini+1*sign(idx_fin-idx_ini)))
    |     y_ini_1 = y_ini
    |     y_fin_1 = perfil(idx_ini+1*sign(idx_fin-idx_ini))
    |     x_ini_1 = x_ini
    |     x_fin_1 = x_ini
    |     t_v_y_1 = (abs(y_fin_1-y_ini_1)/vh_max)+vh_max/ah_max;
    | 
    | else
    |     y_ini_1 = y_ini
    |     y_fin_1 = y_ini
    | 
    |     t_v_y_1 = 0.1
    |     x_ini_1 = x_ini
    |     x_fin_1 = x_ini
    | end
    | 
    | %% Trayecto 2: Parabola/Arco Ascendente
    | y_ini_2 = y_fin_1
    | x_ini_2 = x_fin_1
    | 
    | % Buscamos altura maxima de obstaculo
    | [y_max_obs, idx_max_obs] = max(perfil_rec)
    | y_fin_2 = y_max_obs+10
    | x_fin_2 = 2.44*(idx_ini+idx_max_obs*sign(idx_fin-idx_ini))-30 % -----------------------JUANI---------------------------------
    | 
    | t_v_y_2 = t_v_y_1+(abs(y_fin_2-y_ini_2)/vh_max)+vh_max/ah_max;
    | t_v_x_2 = t_v_y_1+(abs(x_fin_2-x_ini_2)/vt_max)+vt_max/at_max;
    | 
    | 
    | 
    | %% Trayecto 3: Parabola/Arco Descendente
    | y_ini_3 = y_fin_2
    | x_ini_3 = x_fin_2
    | x_fin_3 = x_fin
    | 
    | % Revisamos los alrededores del final para evitar colisiones
    | if (y_fin <= perfil(idx_fin+1*sign(idx_fin-idx_ini)))
    |     y_fin_3 = perfil(idx_fin+1*sign(idx_fin-idx_ini))
    | else
    |     y_fin_3 = y_fin
    | end
    | 
    | t_v_y_3 = t_v_y_2+(abs(y_fin_3-y_ini_3)/vh_max)+vh_max/ah_max;
    | t_v_x_3 = t_v_x_2+(abs(x_fin_3-x_ini_3)/vt_max)+vt_max/at_max;
    | 
    | 
    | t_hitos_y = [0, t_v_y_1, t_v_y_2, t_v_y_3]
    | length(t_hitos_y);
    | t_hitos_x = [0, t_v_y_1, t_v_x_2, t_v_x_3]
    | length(t_hitos_x);
    | x_hitos = [x_ini, x_fin_1, x_fin_2, x_fin_3]
    | length(x_hitos);
    | y_hitos = [y_ini, y_fin_1, y_fin_2, y_fin_3]
    | length(y_hitos);
    | t_v_max = max(t_v_y_3,t_v_x_3)
    | t_vec_new = 0:Ts:t_v_max;
    | length(t_vec_new)
    | 
    | x_ref = minjerkpolytraj(x_hitos, t_hitos_x, length(t_vec_new));
    | y_ref = minjerkpolytraj(y_hitos, t_hitos_y, length(t_vec_new));
    | 
    | % Convertimos la referencia a lh
    | y_ref=45-y_ref;
    | 
    | consignas = zeros(5,length(t_vec_new));
    | 
    | 
    | vx_ref = gradient(x_ref,Ts);
    | vy_ref = gradient(y_ref,Ts);
    | ax_ref = gradient(vx_ref,Ts);
    | sax_ref = gradient(ax_ref,Ts);
    | 
    | 
    | consignas(1,:) = x_ref;
    | consignas(2,:) = y_ref;
    | consignas(3,:) = vx_ref;
    | consignas(4,:) = vy_ref;
    | consignas(5,:) = ax_ref;
    | 
    | end

== stateflow chart PLANTA_COMPLETA/Nivel 0 - Seguridad o Proteccion ==
  settings: updateMethod=DISCRETE  sampleTime=T_s0
  state CONTROL_SEGURIDAD
    state Verificacion
      entry:
      EmergenciaNivel = 0;
      BRK_t = 1;
      BRK_h = 1;
      BRK_hE = 1;
      cont=0;
      state VERIFICA_WATCHDOG [parallel]
        entry:
        cont = 0;
        settings: executionOrder=1
        state ALIVE
          entry:
          cont = 0;
        state WAIT
        state EMERGENCIA_N1
          entry:
          EmergenciaNivel = 1;
        state CONTADOR
          entry:
          cont = cont + 1;
        (default) -> CONTROL_SEGURIDAD.Verificacion.VERIFICA_WATCHDOG.WAIT
        CONTROL_SEGURIDAD.Verificacion.VERIFICA_WATCHDOG.WAIT -> ALIVE [order 3] : [hasChanged(alive)]
        CONTROL_SEGURIDAD.Verificacion.VERIFICA_WATCHDOG.WAIT -> CONTROL_SEGURIDAD.Verificacion.VERIFICA_WATCHDOG.EMERGENCIA_N1 [order 1] : [cont >= 5]
        ALIVE -> CONTROL_SEGURIDAD.Verificacion.VERIFICA_WATCHDOG.WAIT : [true]
        CONTADOR -> CONTROL_SEGURIDAD.Verificacion.VERIFICA_WATCHDOG.WAIT : [true]
        CONTROL_SEGURIDAD.Verificacion.VERIFICA_WATCHDOG.WAIT -> CONTADOR [order 2] : after(1,sec)
      state VERIFICA_FIN_CARRERA [parallel]
        settings: executionOrder=3
        state EMERGENCIA_N2
          entry:
          EmergenciaNivel = 2;
        state WAIT
        state EMERGENCIA_N3
          entry:
          EmergenciaNivel = 3;
        CONTROL_SEGURIDAD.Verificacion.VERIFICA_FIN_CARRERA.WAIT -> CONTROL_SEGURIDAD.Verificacion.VERIFICA_FIN_CARRERA.EMERGENCIA_N2 [order 1] : [FCE_SUP || FCE_INF]
        (default) -> CONTROL_SEGURIDAD.Verificacion.VERIFICA_FIN_CARRERA.WAIT
        CONTROL_SEGURIDAD.Verificacion.VERIFICA_FIN_CARRERA.WAIT -> EMERGENCIA_N3 [order 2] : [FCE_DER || FCE_IZQ]
      state VERIFICA_PULSADOR [parallel]
        settings: executionOrder=2
        state WAIT
        state EMERGENCIA_N1
          entry:
          EmergenciaNivel = 1;
        (default) -> CONTROL_SEGURIDAD.Verificacion.VERIFICA_PULSADOR.WAIT
        CONTROL_SEGURIDAD.Verificacion.VERIFICA_PULSADOR.WAIT -> CONTROL_SEGURIDAD.Verificacion.VERIFICA_PULSADOR.EMERGENCIA_N1 : [PulsadorEmergecia == 1]
      state VERIFICA_SOBREVELOCIDAD [parallel]
        settings: executionOrder=4
        state WAIT
        state EMERGENCIA_N2
          entry:
          EmergenciaNivel = 2;
        (default) -> CONTROL_SEGURIDAD.Verificacion.VERIFICA_SOBREVELOCIDAD.WAIT
        CONTROL_SEGURIDAD.Verificacion.VERIFICA_SOBREVELOCIDAD.WAIT -> CONTROL_SEGURIDAD.Verificacion.VERIFICA_SOBREVELOCIDAD.EMERGENCIA_N2 : [ dlh>= 1.15*v_max_izaje]
    state Emergencia_TOTAL
      entry:
      BRK_t = 0;
      BRK_h = 0;
      BRK_hE = 0;
    state Emergencia_IZAJE
      entry:
      BRK_h = 0;
      BRK_hE = 0;
    state Emergencia_CARRO
      entry:
      BRK_t = 0;
    (default) -> Verificacion
    Emergencia_TOTAL -> Verificacion : [OK]
    Verificacion -> Emergencia_TOTAL [order 1] : [EmergenciaNivel == 1]
    Emergencia_IZAJE -> Verificacion : [OK]
    Verificacion -> Emergencia_IZAJE [order 2] : [EmergenciaNivel == 2]
    Emergencia_CARRO -> Verificacion : [OK]
    Verificacion -> Emergencia_CARRO [order 3] : [EmergenciaNivel == 3]
  data: alive input; BRK_h output; BRK_t output; FCE_DER input; FCE_IZQ input; FCE_INF input; FCE_SUP input; PulsadorEmergecia input; cont local; v_max_izaje input; dlh input; EmergenciaNivel output int8 =0; OK input; BRK_hE output

== matlab function PLANTA_COMPLETA/sensor ==
  data: y0_array input; distancia output; index input; Yt0 parameter
function distancia= mideDistancia(y0_array,index, Yt0)


if (index>0 && index<=32)
    distancia = Yt0-y0_array(index);
else
   distancia = Yt0;
end

== matlab function PLANTA_COMPLETA/Nivel 2 - Control Regulatorio/Controlador de balanceo/MATLAB Function ==
  data: xt0 input; Kp output; vt0 input; th0 input; w0 input; Ftw0 input; Mt0 input; ml0 input; l0 input; bt0 input; g0 input; Kd output
function [Kp, Kd] = jacob(xt0,vt0,th0,w0,Ftw0,Mt0,ml0,l0,bt0,g0)

syms xt vt th w Ftw real
syms Mt ml l bt g_sym real

%%Linealizacion Jacobiana 

% Estados y entrada
x = [xt; vt; th; w];
u = Ftw;

% Definiciones auxiliares
Dx  = Mt + ml*sin(th)^2;
Nx = Ftw - bt*vt + ml*l*w^2*sin(th) + ml*g_sym*sin(th)*cos(th);
Nth = -(Mt+ml*sin(th)^2)*g_sym*sin(th)-cos(th)*(Ftw-bt*vt+ml*l*w^2*sin(th)+ml*g_sym*sin(th)*cos(th));
Dth = l*(Mt+ml*sin(th)^2);

% Dinámica
f1 = vt;
f2 = Nx / Dx;
f3 = w;
f4 = Nth / Dth;

f = [f1; f2; f3; f4];

% Jacobianos
A = jacobian(f, x);
B = jacobian(f, u);

% (opcional) simplificación
A = simplify(A);
B = simplify(B);

% Modelo LPV evaluado en el punto de operacion
A0 = subs(A, {xt,vt,th,w,Ftw,Mt,ml,l,bt,g_sym}, {xt0,vt0,th0,w0,Ftw0,Mt0,ml0,l0,bt0,g0});
B0 = subs(B, {xt,vt,th,w,Ftw,Mt,ml,l,bt,g_sym}, {xt0,vt0,th0,w0,Ftw0,Mt0,ml0,l0,bt0,g0});

%% Buscamos la dinamica natural del sistema
% Autovalores de la matriz A0
lambda = eig(double(A0));

% Ordenar por real(lambda) (más cercano a 0 -> dominante)
[~, idx] = sort(real(lambda), 'descend'); % mayor real -> más lento (menos negativo)
lambda_ord = lambda(idx);

% Seleccionar el primer autovalor
lambda_dom = lambda_ord(1);

% Si es complejo (par), buscar su conjugado y calcular wn_la
if imag(lambda_dom) ~= 0
    sigma = real(lambda_dom);
    wd = abs(imag(lambda_dom));
    wn_la = sqrt(sigma^2 + wd^2);
    dseta = -sigma / wn_la;
else
    % polo real dominante
    sigma = real(lambda_dom);   % negativo para estable
    wn_la = abs(sigma);       % uso de |sigma| como medida de velocidad
    dseta = 1;              % no aplica exactamente, placeholder
end

%% Obtencion de Funcion de transferencia
syms Kp Kd s real

Gc = Kp+Kd*s;

% Selección de salida y vector que representa la acción de delta-theta
C = [0 1 0 0];            % salida y = delta v_t
a_theta = A0(:,3);        % influencia de delta theta como "entrada"

%Para encontrar la funcion de transferencia
SI_A0 = s*eye(4) - A0;
Gp = simplify( C * inv(SI_A0)* B(:,1));  % TF de la planta

% Separar numerador y denominador simbólicos (opcional)
% [numG, denG] = numden(Gp);
% numG = simplify(expand(numG));
% denG = simplify(expand(denG));

% 
% Gct = (1.7024e+04)/(s^2)+(2.2754e+04)/s+(1.0849e+04);
% Gct = simplify(Gct);
% 
% Gcb = Gp/(1+Gct*Gc*Gp); 

Gcb = Gp/(1+Gc*Gp)
Gcb = simplify(Gcb);
[~, denGcb] = numden(Gcb);
denGcb = expand(denGcb);

%% Diseño por amortiguamiento crítico
% Usamos una wn mayor a la de lazo abierto
wn = 1.5*wn_la;

% Polinomio dominante de segundo orden crítico
P_dom = s^2 + 2*wn*s + wn^2;

% Polos no dominantes (rápidos)
alpha = 5*wn;
beta = 6*wn;
P_des = expand(P_dom * (s + alpha) * (s + beta));

% Polinomio del lazo cerrado
P_lc = denGcb;

% % Igualación de coeficientes
% Pdiff = (expand(D_lc - D_des));
% coeffs_vec = coeffs(Pdiff, s);
% eqs = coeffs_vec == 0;

% Forma robusta: extraer polinomio en vector
% [~,D_des_p] = numden(D_des);
% poly_des = expand(D_des);

% Igualación por coeficientes (grado 4 -> 5 ecuaciones)
coeffs_lc = coeffs(P_lc,s,'All');
coeffs_des = coeffs(P_des, s, 'All');

% alinear longitudes rellenando con ceros si es necesario
nL = length(coeffs_lc); nD = length(coeffs_des);
n = max(nL, nD);
coeffs_lc = [zeros(1,n-nL), coeffs_lc];
coeffs_des = [zeros(1,n-nD), coeffs_des];

% formar sistema de ecuaciones (vectorial)
eqs = coeffs_lc - coeffs_des;
eqs = simplify(eqs);           % ecuaciones simbólicas

% Resolver simbólicamente Kp, Kd
sol = solve(eqs, [Kp Kd], 'Real', true);

% recoger soluciones posibles
Kp_sol = sol.Kp;
Kd_sol = sol.Kd;

% % Si solve devuelve múltiples soluciones, filtrar:
% found = false;
% Kp = NaN; Kd = NaN; wn = NaN;
%     for i = 1:length(wn_sym)
%         try
%             wn_i = double(wn_sym(i));
%             Kp_i = double(Kp_sym(i));
%             Kd_i = double(Kd_sym(i));
%         catch
%             continue;
%         end
%         if ~isreal(wn_i) || wn_i <= 0 || ~isreal(Kp_i) || ~isreal(Kd_i)
%             continue;
%         end
%         % comprobar estabilidad del lazo cerrado
%         poly_lc_sub = double(subs(poly_lc, {Kp,Kd,wn}, {Kp_i,Kd_i,wn_i}));
%         % opcional: comprobar raices todas en LHP
%         coeff_vec = sym2poly(poly_lc_sub);
%         if isempty(coeff_vec)
%             continue;
%         end
%         rts = roots(coeff_vec);
%         if all(real(rts) < 0)
%             Kp = Kp_i; Kd = Kd_i; wn = wn_i;
%             found = true;
%         end
%     end
% 
%     if ~found
%         warning('No se encontró solución válida para Kp,Kd,wn con los criterios dados.');
%     end

end

== stateflow chart PLANTA_COMPLETA/Enclavamiento ==
  state Espera
  state Cambiar
    entry:
    output=(~output);
  (default) -> Espera
  Espera -> Cambiar : [input]
  Cambiar -> Espera : [input==0]
  data: input input; output output boolean =false

== matlab function PLANTA_COMPLETA/Calculo ==
  data: masas_array input; Mc_X output; index input
function Mc_X= calcula_Mc_X(masas_array,index)
if (index>0 && index<=32)
    Mc_X =masas_array(index);
else
    Mc_X=0;
end

== stateflow chart PLANTA_COMPLETA/Enclavamiento1 ==
  state Espera
  state Cambiar
    entry:
    output=(~output);
  (default) -> Espera
  Espera -> Cambiar : [input]
  Cambiar -> Espera : [input==0]
  data: input input; output output boolean =false

== matlab function PLANTA_COMPLETA/Velocidad max izaje ==
  data: M_l input; dxt_max output
function dxt_max = fcn(M_l)

Pnom=956.15e3; %Potencia nominal motor
g= 9.80665; %Acel gravitatoria

if (M_l>=65000)
    dxt_max = 1.5; %1.5 m/s
elseif (32500<=M_l)&&(M_l<65000)
    dxt_max = Pnom/(M_l*g);
elseif (M_l<32500)
    dxt_max=3; %3 m/s
else
    dxt_max = 1.5;

end

== matlab function PLANTA_COMPLETA/PLANTA/Masa de contenedor (A partir de posicion x_l)/Calculo ==
  data: masas_array input; Mc_X output; index input
function Mc_X= calcula_Mc_X(masas_array,index)

if (index>0 && index<=32)
    Mc_X =masas_array(index);
else
    Mc_X=0;

end

== matlab function PLANTA_COMPLETA/Actualizar perfil/Enabled Subsystem/Actualiza perfil ==
  data: index input; y0_actualizado output; y0 input; Hc input
function y0_actualizado = fcn(index,y0,Hc)
y0_anterior=y0;
if (abs(index)>0 && abs(index)<=32)
y0_anterior(abs(index))=y0_anterior(abs(index))+Hc*sign(index);
y0_actualizado=y0_anterior;
else
y0_actualizado=y0;
end
